simulink model "stewart_platform"  (R2019b)
settings: configuration reference "conf_simscape" (kept outside this file)
undefined symbols (not defined in the file): stewart, X, Y, Z
libraries: sm_lib x20, nesl_utility x1
settings Model: Creator=thomas  LastModifiedBy=thomas
settings ConfigSetRef: SourceName=conf_simscape  SourceLocation=Base Workspace

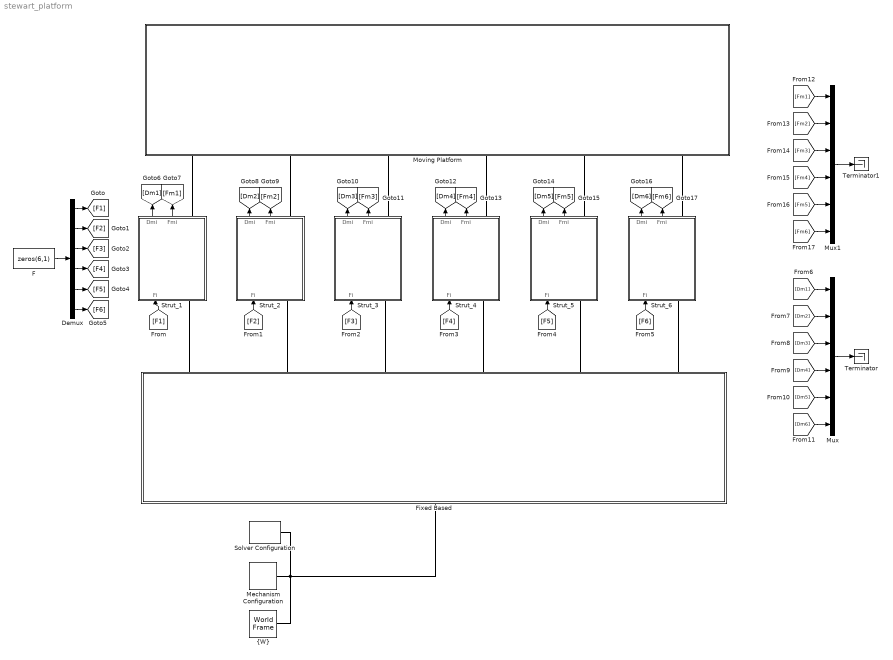
== system stewart_platform ==
  Demux : Demux  Outputs=6
  F : Constant  Value=zeros(6,1)
  Fixed Based : Subsystem
  Mechanism Configuration : sm_lib/Utilities/Mechanism Configuration  UniformGravity=Constant  GravityVector=[0 0 0]  GravityUnits=m/s^2  LinearizationDelta=0.001
  Moving Platform : Subsystem
  Mux : Mux  Inputs=6
  Mux1 : Mux  Inputs=6
  Solver Configuration : nesl_utility/Solver Configuration  PhysicalDomain=network_engine_domain  SubClassName=solver  LeftPortType=input  RightPortType=generic  Tones=[]  Harmonics=[]  SimulateNoise=off  Profile=off  UseLocalSampling=off  EnableSwitchedLinearOptims=on  FrequencyDomain=off  UseCCode=off  RelTol=0.001  AbsTol=1e-06  MinStep=1e-09  ToWorkspace=off  RevertToSquareIcSolve=off  NumHomotopyIterations=100  PhasorMode=off  PhasorModeNumHarmonics=1  DoDC=off  ResidualTolerance=1e-09  UseLocalSolver=off  LocalSolverChoice=NE_BACKWARD_EULER_ADVANCER  LocalSolverSampleTime=0.001  DoFixedCost=off  MaxNonlinIter=3  MaxModeIter=2  LinearAlgebra=auto  EquationFormulation=NE_TIME_EF  DelaysMemoryBudget=1024  AutomaticFiltering=on  FilteringTimeConstant=0.001  PartitionStorageMethod=AS_NEEDED  PartitionMemoryBudget=1024  PartitionMethod=ROBUST
  Strut_1 : Subsystem
      mask init:
      | i=1;
  Strut_2 : Subsystem
      mask init:
      | i=2;
  Strut_3 : Subsystem
      mask init:
      | i=3;
  Strut_4 : Subsystem
      mask init:
      | i=4;
  Strut_5 : Subsystem
      mask init:
      | i=5;
  Strut_6 : Subsystem
      mask init:
      | i=6;
  Terminator : Terminator
  Terminator1 : Terminator
  "{W}" : sm_lib/Frames and Transforms/World Frame
  wires:
  F/1 -> Demux/1
  Demux/1 -> [F1]
  Demux/2 -> [F2]
  [F1] -> Strut_1/1(Fi)
  Demux/3 -> [F3]
  Demux/4 -> [F4]
  Demux/5 -> [F5]
  Demux/6 -> [F6]
  [F2] -> Strut_2/1(Fi)
  [F4] -> Strut_4/1(Fi)
  [F5] -> Strut_5/1(Fi)
  [F6] -> Strut_6/1(Fi)
  Strut_1/1(Dmi) -> [Dm1]
  Strut_1/2(Fmi) -> [Fm1]
  Strut_2/2(Fmi) -> [Fm2]
  [F3] -> Strut_3/1(Fi)
  Strut_2/1(Dmi) -> [Dm2]
  Strut_3/1(Dmi) -> [Dm3]
  Strut_3/2(Fmi) -> [Fm3]
  Strut_4/1(Dmi) -> [Dm4]
  Strut_4/2(Fmi) -> [Fm4]
  Strut_5/1(Dmi) -> [Dm5]
  Strut_5/2(Fmi) -> [Fm5]
  Strut_6/1(Dmi) -> [Dm6]
  Strut_6/2(Fmi) -> [Fm6]
  [Dm2] -> Mux/2
  [Dm1] -> Mux/1
  [Dm3] -> Mux/3
  [Dm4] -> Mux/4
  [Dm5] -> Mux/5
  [Dm6] -> Mux/6
  Mux/1 -> Terminator/1
  [Fm6] -> Mux1/6
  [Fm5] -> Mux1/5
  [Fm1] -> Mux1/1
  [Fm2] -> Mux1/2
  [Fm3] -> Mux1/3
  [Fm4] -> Mux1/4
  Mux1/1 -> Terminator1/1
  connections:
  "{W}"/RConn1 -- Fixed Based/LConn1 -- Solver Configuration/RConn1 -- Mechanism Configuration/RConn1
  Fixed Based/RConn2 -- Strut_2/LConn1
  Fixed Based/RConn3 -- Strut_3/LConn1
  Fixed Based/RConn4 -- Strut_4/LConn1
  Fixed Based/RConn5 -- Strut_5/LConn1
  Fixed Based/RConn6 -- Strut_6/LConn1
  Strut_2/RConn1 -- Moving Platform/LConn2
  Strut_3/RConn1 -- Moving Platform/LConn3
  Strut_4/RConn1 -- Moving Platform/LConn4
  Strut_5/RConn1 -- Moving Platform/LConn5
  Strut_6/RConn1 -- Moving Platform/LConn6
  Strut_1/LConn1 -- Fixed Based/RConn1
  Strut_1/RConn1 -- Moving Platform/LConn1

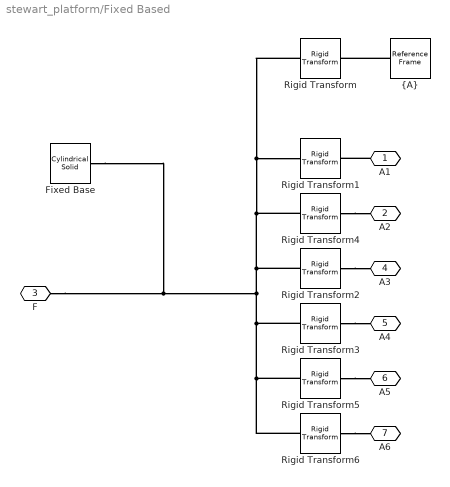
== system stewart_platform/Fixed Based ==
  Fixed Base : sm_lib/Body Elements/Cylindrical Solid  GraphicAmbientColor=[0.15 0.15 0.15 1.0]  BasedOnType=Density  CenterOfMass=[0 0 0]  CenterOfMassUnits=m  GraphicDiffuseColor=[0.5 0.5 0.5]  CylinderLength=10e-3  CylinderLengthUnits=m  CylinderRadius=100e-3  CylinderRadiusUnits=m  Density=1000  DensityUnits=kg/m^3  DoExposeReferenceFrame=off  GraphicEmissiveColor=[0.0 0.0 0.0 1.0]  ExportEntireGeometry=off  SerializedFrames=<Frames><Frame><Id>Frame1</Id><Value><Name>{F}</Name><Origin><Source>GeometricFeature</Source><FeatureName>bottom surface</FeatureName></Origin><PrimaryAxis><DefinedDirection>+Z</DefinedDirection><Source>ReferenceFrame</Source><SourceDirection>+Z</SourceDirection><FeatureName></FeatureName></PrimaryAxis><SecondaryAxis><DefinedDirection>+X</DefinedDirection><Source>ReferenceFrame</Source><SourceDirection>+X</SourceDirection><FeatureName></FeatureName></SecondaryAxis></Value></Frame></Frames>  MarkerShape=Sphere  MarkerSize=10  GraphicType=FromGeometry  InertiaType=CalculateFromGeometry  Mass=1  MassUnits=kg  MomentsOfInertia=[1 1 1]  MomentsOfInertiaUnits=kg*m^2  GraphicOpacity=1.0  ProductsOfInertia=[0 0 0]  ProductsOfInertiaUnits=kg*m^2  GraphicShininess=75  GraphicSpecularColor=[0.5 0.5 0.5 1.0]  GraphicVisPropType=SimpleVisualProperties
  Rigid Transform : sm_lib/Frames and Transforms/Rigid Transform  TranslationMethod=Cartesian  TranslationStandardOffset=0  TranslationLengthUnit=m  TranslationStandardAxis=+Z  TranslationCartesianOffset=stewart.FO_A  TranslationROffset=0  TranslationROffsetUnits=m  TranslationZOffset=0  TranslationZOffsetUnits=m  TranslationThetaOffset=0  TranslationThetaOffsetUnits=deg  RotationMethod=None  RotationAngleUnits=deg  RotationStandardAxis=+Z  RotationAngle=0.0  RotationArbitraryAxis=[0 0 1]  FollAlignAxisA=+X  BaseAlignAxisA=+Y  FollAlignAxisB=+Y  BaseAlignAxisB=+Z  RotationSequenceAxes=FollowerAxes  RotationSequence=XYX  RotationSequenceAngles=[0 0 0]  RotationSequenceAnglesUnits=deg  RotationMatrix=[1 0 0; 0 1 0; 0 0 1]
  Rigid Transform1 : sm_lib/Frames and Transforms/Rigid Transform  TranslationMethod=Cartesian  TranslationStandardOffset=0  TranslationLengthUnit=m  TranslationStandardAxis=+Z  TranslationCartesianOffset=stewart.Fa(:, 1)  TranslationROffset=0  TranslationROffsetUnits=m  TranslationZOffset=0  TranslationZOffsetUnits=m  TranslationThetaOffset=0  TranslationThetaOffsetUnits=deg  RotationMethod=RotationMatrix  RotationAngleUnits=deg  RotationStandardAxis=+Z  RotationAngle=0.0  RotationArbitraryAxis=[0 0 1]  FollAlignAxisA=+X  BaseAlignAxisA=+Y  FollAlignAxisB=+Y  BaseAlignAxisB=+Z  RotationSequenceAxes=FollowerAxes  RotationSequence=XYX  RotationSequenceAngles=[0 0 0]  RotationSequenceAnglesUnits=deg  RotationMatrix=stewart.FRa(:, :, 1)
  Rigid Transform2 : sm_lib/Frames and Transforms/Rigid Transform  TranslationMethod=Cartesian  TranslationStandardOffset=0  TranslationLengthUnit=m  TranslationStandardAxis=+Z  TranslationCartesianOffset=stewart.Fa(:, 3)  TranslationROffset=0  TranslationROffsetUnits=m  TranslationZOffset=0  TranslationZOffsetUnits=m  TranslationThetaOffset=0  TranslationThetaOffsetUnits=deg  RotationMethod=RotationMatrix  RotationAngleUnits=deg  RotationStandardAxis=+Z  RotationAngle=0.0  RotationArbitraryAxis=[0 0 1]  FollAlignAxisA=+X  BaseAlignAxisA=+Y  FollAlignAxisB=+Y  BaseAlignAxisB=+Z  RotationSequenceAxes=FollowerAxes  RotationSequence=XYX  RotationSequenceAngles=[0 0 0]  RotationSequenceAnglesUnits=deg  RotationMatrix=stewart.FRa(:, :, 3)
  Rigid Transform3 : sm_lib/Frames and Transforms/Rigid Transform  TranslationMethod=Cartesian  TranslationStandardOffset=0  TranslationLengthUnit=m  TranslationStandardAxis=+Z  TranslationCartesianOffset=stewart.Fa(:, 4)  TranslationROffset=0  TranslationROffsetUnits=m  TranslationZOffset=0  TranslationZOffsetUnits=m  TranslationThetaOffset=0  TranslationThetaOffsetUnits=deg  RotationMethod=RotationMatrix  RotationAngleUnits=deg  RotationStandardAxis=+Z  RotationAngle=0.0  RotationArbitraryAxis=[0 0 1]  FollAlignAxisA=+X  BaseAlignAxisA=+Y  FollAlignAxisB=+Y  BaseAlignAxisB=+Z  RotationSequenceAxes=FollowerAxes  RotationSequence=XYX  RotationSequenceAngles=[0 0 0]  RotationSequenceAnglesUnits=deg  RotationMatrix=stewart.FRa(:, :, 4)
  Rigid Transform4 : sm_lib/Frames and Transforms/Rigid Transform  TranslationMethod=Cartesian  TranslationStandardOffset=0  TranslationLengthUnit=m  TranslationStandardAxis=+Z  TranslationCartesianOffset=stewart.Fa(:, 2)  TranslationROffset=0  TranslationROffsetUnits=m  TranslationZOffset=0  TranslationZOffsetUnits=m  TranslationThetaOffset=0  TranslationThetaOffsetUnits=deg  RotationMethod=RotationMatrix  RotationAngleUnits=deg  RotationStandardAxis=+Z  RotationAngle=0.0  RotationArbitraryAxis=[0 0 1]  FollAlignAxisA=+X  BaseAlignAxisA=+Y  FollAlignAxisB=+Y  BaseAlignAxisB=+Z  RotationSequenceAxes=FollowerAxes  RotationSequence=XYX  RotationSequenceAngles=[0 0 0]  RotationSequenceAnglesUnits=deg  RotationMatrix=stewart.FRa(:, :, 2)
  Rigid Transform5 : sm_lib/Frames and Transforms/Rigid Transform  TranslationMethod=Cartesian  TranslationStandardOffset=0  TranslationLengthUnit=m  TranslationStandardAxis=+Z  TranslationCartesianOffset=stewart.Fa(:, 5)  TranslationROffset=0  TranslationROffsetUnits=m  TranslationZOffset=0  TranslationZOffsetUnits=m  TranslationThetaOffset=0  TranslationThetaOffsetUnits=deg  RotationMethod=RotationMatrix  RotationAngleUnits=deg  RotationStandardAxis=+Z  RotationAngle=0.0  RotationArbitraryAxis=[0 0 1]  FollAlignAxisA=+X  BaseAlignAxisA=+Y  FollAlignAxisB=+Y  BaseAlignAxisB=+Z  RotationSequenceAxes=FollowerAxes  RotationSequence=XYX  RotationSequenceAngles=[0 0 0]  RotationSequenceAnglesUnits=deg  RotationMatrix=stewart.FRa(:, :, 5)
  Rigid Transform6 : sm_lib/Frames and Transforms/Rigid Transform  TranslationMethod=Cartesian  TranslationStandardOffset=0  TranslationLengthUnit=m  TranslationStandardAxis=+Z  TranslationCartesianOffset=stewart.Fa(:, 6)  TranslationROffset=0  TranslationROffsetUnits=m  TranslationZOffset=0  TranslationZOffsetUnits=m  TranslationThetaOffset=0  TranslationThetaOffsetUnits=deg  RotationMethod=RotationMatrix  RotationAngleUnits=deg  RotationStandardAxis=+Z  RotationAngle=0.0  RotationArbitraryAxis=[0 0 1]  FollAlignAxisA=+X  BaseAlignAxisA=+Y  FollAlignAxisB=+Y  BaseAlignAxisB=+Z  RotationSequenceAxes=FollowerAxes  RotationSequence=XYX  RotationSequenceAngles=[0 0 0]  RotationSequenceAnglesUnits=deg  RotationMatrix=stewart.FRa(:, :, 6)
  "{A}" : sm_lib/Frames and Transforms/Reference Frame
  A1 : PMIOPort  Side=Right
  A2 : PMIOPort  Port=2  Side=Right
  F : PMIOPort  Port=3  Side=Left
  A3 : PMIOPort  Port=4  Side=Right
  A4 : PMIOPort  Port=5  Side=Right
  A5 : PMIOPort  Port=6  Side=Right
  A6 : PMIOPort  Port=7  Side=Right
  connections:
  Rigid Transform4/RConn1 -- A2/RConn1
  "{A}"/RConn1 -- Rigid Transform/RConn1
  A1/RConn1 -- Rigid Transform1/RConn1
  Rigid Transform/LConn1 -- Rigid Transform1/LConn1 -- Rigid Transform6/LConn1 -- Rigid Transform5/LConn1 -- Rigid Transform3/LConn1 -- F/RConn1 -- Fixed Base/LConn1 -- Rigid Transform2/LConn1 -- Rigid Transform4/LConn1
  Rigid Transform2/RConn1 -- A3/RConn1
  Rigid Transform3/RConn1 -- A4/RConn1
  Rigid Transform5/RConn1 -- A5/RConn1
  Rigid Transform6/RConn1 -- A6/RConn1

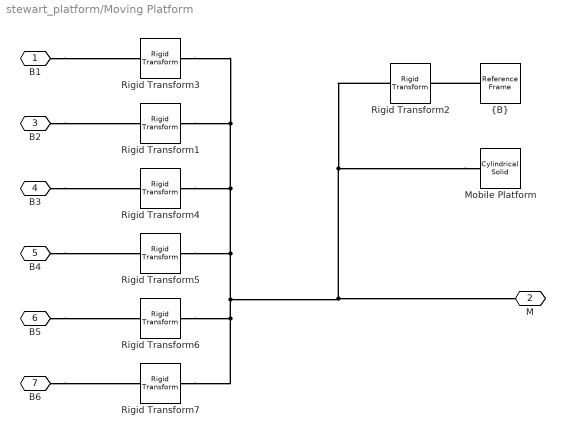
== system stewart_platform/Moving Platform ==
  Mobile Platform : sm_lib/Body Elements/Cylindrical Solid  GraphicAmbientColor=[0.15 0.15 0.15 1.0]  BasedOnType=Density  CenterOfMass=[0 0 0]  CenterOfMassUnits=m  GraphicDiffuseColor=[0.5 0.5 0.5]  CylinderLength=10e-3  CylinderLengthUnits=m  CylinderRadius=100e-3  CylinderRadiusUnits=m  Density=1000  DensityUnits=kg/m^3  DoExposeReferenceFrame=off  GraphicEmissiveColor=[0.0 0.0 0.0 1.0]  ExportEntireGeometry=off  SerializedFrames=<Frames><Frame><Id>Frame1</Id><Value><Name>{M}</Name><Origin><Source>GeometricFeature</Source><FeatureName>top surface</FeatureName></Origin><PrimaryAxis><DefinedDirection>+Z</DefinedDirection><Source>ReferenceFrame</Source><SourceDirection>+Z</SourceDirection><FeatureName></FeatureName></PrimaryAxis><SecondaryAxis><DefinedDirection>+X</DefinedDirection><Source>ReferenceFrame</Source><SourceDirection>+X</SourceDirection><FeatureName></FeatureName></SecondaryAxis></Value></Frame></Frames>  MarkerShape=Sphere  MarkerSize=10  GraphicType=FromGeometry  InertiaType=CalculateFromGeometry  Mass=1  MassUnits=kg  MomentsOfInertia=[1 1 1]  MomentsOfInertiaUnits=kg*m^2  GraphicOpacity=1.0  ProductsOfInertia=[0 0 0]  ProductsOfInertiaUnits=kg*m^2  GraphicShininess=75  GraphicSpecularColor=[0.5 0.5 0.5 1.0]  GraphicVisPropType=SimpleVisualProperties
  Rigid Transform1 : sm_lib/Frames and Transforms/Rigid Transform  TranslationMethod=Cartesian  TranslationStandardOffset=0  TranslationLengthUnit=m  TranslationStandardAxis=+Z  TranslationCartesianOffset=stewart.Mb(:, 2)  TranslationROffset=0  TranslationROffsetUnits=m  TranslationZOffset=0  TranslationZOffsetUnits=m  TranslationThetaOffset=0  TranslationThetaOffsetUnits=deg  RotationMethod=RotationMatrix  RotationAngleUnits=deg  RotationStandardAxis=+Z  RotationAngle=0.0  RotationArbitraryAxis=[0 0 1]  FollAlignAxisA=+X  BaseAlignAxisA=+Y  FollAlignAxisB=+Y  BaseAlignAxisB=+Z  RotationSequenceAxes=FollowerAxes  RotationSequence=XYX  RotationSequenceAngles=[0 0 0]  RotationSequenceAnglesUnits=deg  RotationMatrix=stewart.MRb(:, :, 2)
  Rigid Transform2 : sm_lib/Frames and Transforms/Rigid Transform  TranslationMethod=Cartesian  TranslationStandardOffset=0  TranslationLengthUnit=m  TranslationStandardAxis=+Z  TranslationCartesianOffset=stewart.MO_B  TranslationROffset=0  TranslationROffsetUnits=m  TranslationZOffset=0  TranslationZOffsetUnits=m  TranslationThetaOffset=0  TranslationThetaOffsetUnits=deg  RotationMethod=None  RotationAngleUnits=deg  RotationStandardAxis=+Z  RotationAngle=0.0  RotationArbitraryAxis=[0 0 1]  FollAlignAxisA=+X  BaseAlignAxisA=+Y  FollAlignAxisB=+Y  BaseAlignAxisB=+Z  RotationSequenceAxes=FollowerAxes  RotationSequence=XYX  RotationSequenceAngles=[0 0 0]  RotationSequenceAnglesUnits=deg  RotationMatrix=[1 0 0; 0 1 0; 0 0 1]
  Rigid Transform3 : sm_lib/Frames and Transforms/Rigid Transform  TranslationMethod=Cartesian  TranslationStandardOffset=0  TranslationLengthUnit=m  TranslationStandardAxis=+Z  TranslationCartesianOffset=stewart.Mb(:, 1)  TranslationROffset=0  TranslationROffsetUnits=m  TranslationZOffset=0  TranslationZOffsetUnits=m  TranslationThetaOffset=0  TranslationThetaOffsetUnits=deg  RotationMethod=RotationMatrix  RotationAngleUnits=deg  RotationStandardAxis=+Z  RotationAngle=0.0  RotationArbitraryAxis=[0 0 1]  FollAlignAxisA=+X  BaseAlignAxisA=+Y  FollAlignAxisB=+Y  BaseAlignAxisB=+Z  RotationSequenceAxes=FollowerAxes  RotationSequence=XYX  RotationSequenceAngles=[0 0 0]  RotationSequenceAnglesUnits=deg  RotationMatrix=stewart.MRb(:, :, 1)
  Rigid Transform4 : sm_lib/Frames and Transforms/Rigid Transform  TranslationMethod=Cartesian  TranslationStandardOffset=0  TranslationLengthUnit=m  TranslationStandardAxis=+Z  TranslationCartesianOffset=stewart.Mb(:, 3)  TranslationROffset=0  TranslationROffsetUnits=m  TranslationZOffset=0  TranslationZOffsetUnits=m  TranslationThetaOffset=0  TranslationThetaOffsetUnits=deg  RotationMethod=RotationMatrix  RotationAngleUnits=deg  RotationStandardAxis=+Z  RotationAngle=0.0  RotationArbitraryAxis=[0 0 1]  FollAlignAxisA=+X  BaseAlignAxisA=+Y  FollAlignAxisB=+Y  BaseAlignAxisB=+Z  RotationSequenceAxes=FollowerAxes  RotationSequence=XYX  RotationSequenceAngles=[0 0 0]  RotationSequenceAnglesUnits=deg  RotationMatrix=stewart.MRb(:, :, 3)
  Rigid Transform5 : sm_lib/Frames and Transforms/Rigid Transform  TranslationMethod=Cartesian  TranslationStandardOffset=0  TranslationLengthUnit=m  TranslationStandardAxis=+Z  TranslationCartesianOffset=stewart.Mb(:, 4)  TranslationROffset=0  TranslationROffsetUnits=m  TranslationZOffset=0  TranslationZOffsetUnits=m  TranslationThetaOffset=0  TranslationThetaOffsetUnits=deg  RotationMethod=RotationMatrix  RotationAngleUnits=deg  RotationStandardAxis=+Z  RotationAngle=0.0  RotationArbitraryAxis=[0 0 1]  FollAlignAxisA=+X  BaseAlignAxisA=+Y  FollAlignAxisB=+Y  BaseAlignAxisB=+Z  RotationSequenceAxes=FollowerAxes  RotationSequence=XYX  RotationSequenceAngles=[0 0 0]  RotationSequenceAnglesUnits=deg  RotationMatrix=stewart.MRb(:, :, 4)
  Rigid Transform6 : sm_lib/Frames and Transforms/Rigid Transform  TranslationMethod=Cartesian  TranslationStandardOffset=0  TranslationLengthUnit=m  TranslationStandardAxis=+Z  TranslationCartesianOffset=stewart.Mb(:, 5)  TranslationROffset=0  TranslationROffsetUnits=m  TranslationZOffset=0  TranslationZOffsetUnits=m  TranslationThetaOffset=0  TranslationThetaOffsetUnits=deg  RotationMethod=RotationMatrix  RotationAngleUnits=deg  RotationStandardAxis=+Z  RotationAngle=0.0  RotationArbitraryAxis=[0 0 1]  FollAlignAxisA=+X  BaseAlignAxisA=+Y  FollAlignAxisB=+Y  BaseAlignAxisB=+Z  RotationSequenceAxes=FollowerAxes  RotationSequence=XYX  RotationSequenceAngles=[0 0 0]  RotationSequenceAnglesUnits=deg  RotationMatrix=stewart.MRb(:, :, 5)
  Rigid Transform7 : sm_lib/Frames and Transforms/Rigid Transform  TranslationMethod=Cartesian  TranslationStandardOffset=0  TranslationLengthUnit=m  TranslationStandardAxis=+Z  TranslationCartesianOffset=stewart.Mb(:, 6)  TranslationROffset=0  TranslationROffsetUnits=m  TranslationZOffset=0  TranslationZOffsetUnits=m  TranslationThetaOffset=0  TranslationThetaOffsetUnits=deg  RotationMethod=RotationMatrix  RotationAngleUnits=deg  RotationStandardAxis=+Z  RotationAngle=0.0  RotationArbitraryAxis=[0 0 1]  FollAlignAxisA=+X  BaseAlignAxisA=+Y  FollAlignAxisB=+Y  BaseAlignAxisB=+Z  RotationSequenceAxes=FollowerAxes  RotationSequence=XYX  RotationSequenceAngles=[0 0 0]  RotationSequenceAnglesUnits=deg  RotationMatrix=stewart.MRb(:, :, 6)
  "{B}" : sm_lib/Frames and Transforms/Reference Frame
  B1 : PMIOPort  Side=Left
  M : PMIOPort  Port=2  Side=Right
  B2 : PMIOPort  Port=3  Side=Left
  B3 : PMIOPort  Port=4  Side=Left
  B4 : PMIOPort  Port=5  Side=Left
  B5 : PMIOPort  Port=6  Side=Left
  B6 : PMIOPort  Port=7  Side=Left
  connections:
  Mobile Platform/LConn1 -- Rigid Transform5/LConn1 -- Rigid Transform4/LConn1 -- Rigid Transform1/LConn1 -- Rigid Transform3/LConn1 -- Rigid Transform6/LConn1 -- Rigid Transform7/LConn1 -- M/RConn1 -- Rigid Transform2/LConn1
  B1/RConn1 -- Rigid Transform3/RConn1
  "{B}"/RConn1 -- Rigid Transform2/RConn1
  B2/RConn1 -- Rigid Transform1/RConn1
  B3/RConn1 -- Rigid Transform4/RConn1
  B4/RConn1 -- Rigid Transform5/RConn1
  B5/RConn1 -- Rigid Transform6/RConn1
  B6/RConn1 -- Rigid Transform7/RConn1

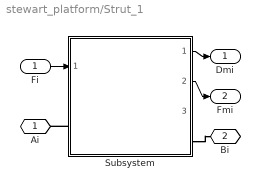
== system stewart_platform/Strut_1 ==
  Fi : Inport
  Subsystem : Subsystem  VariantControl=with_sensors  ReferencedSubsystem=stewart_strut
  Ai : PMIOPort  Side=Left
  Bi : PMIOPort  Port=2  Side=Right
  Dmi : Outport
  Fmi : Outport  Port=2
  wires:
  Subsystem/1 -> Dmi/1
  Subsystem/2 -> Fmi/1
  Fi/1 -> Subsystem/1
  connections:
  Subsystem/LConn1 -- Ai/RConn1
  Subsystem/RConn1 -- Bi/RConn1

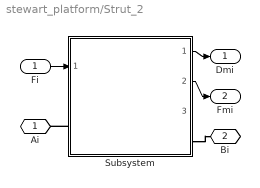
== system stewart_platform/Strut_2 ==
  Fi : Inport
  Subsystem : Subsystem  VariantControl=with_sensors  ReferencedSubsystem=stewart_strut
  Ai : PMIOPort  Side=Left
  Bi : PMIOPort  Port=2  Side=Right
  Dmi : Outport
  Fmi : Outport  Port=2
  wires:
  Fi/1 -> Subsystem/1
  Subsystem/2 -> Fmi/1
  Subsystem/1 -> Dmi/1
  connections:
  Subsystem/RConn1 -- Bi/RConn1
  Subsystem/LConn1 -- Ai/RConn1

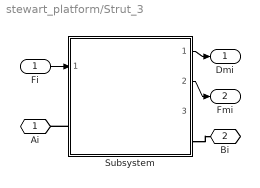
== system stewart_platform/Strut_3 ==
  Fi : Inport
  Subsystem : Subsystem  VariantControl=with_sensors  ReferencedSubsystem=stewart_strut
  Ai : PMIOPort  Side=Left
  Bi : PMIOPort  Port=2  Side=Right
  Dmi : Outport
  Fmi : Outport  Port=2
  wires:
  Subsystem/1 -> Dmi/1
  Subsystem/2 -> Fmi/1
  Fi/1 -> Subsystem/1
  connections:
  Subsystem/LConn1 -- Ai/RConn1
  Subsystem/RConn1 -- Bi/RConn1

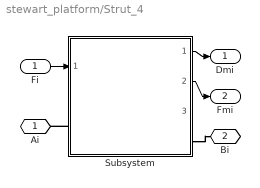
== system stewart_platform/Strut_4 ==
  Fi : Inport
  Subsystem : Subsystem  VariantControl=with_sensors  ReferencedSubsystem=stewart_strut
  Ai : PMIOPort  Side=Left
  Bi : PMIOPort  Port=2  Side=Right
  Dmi : Outport
  Fmi : Outport  Port=2
  wires:
  Fi/1 -> Subsystem/1
  Subsystem/2 -> Fmi/1
  Subsystem/1 -> Dmi/1
  connections:
  Subsystem/RConn1 -- Bi/RConn1
  Subsystem/LConn1 -- Ai/RConn1

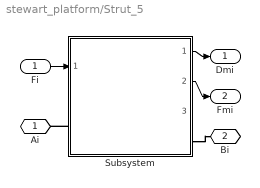
== system stewart_platform/Strut_5 ==
  Fi : Inport
  Subsystem : Subsystem  VariantControl=with_sensors  ReferencedSubsystem=stewart_strut
  Ai : PMIOPort  Side=Left
  Bi : PMIOPort  Port=2  Side=Right
  Dmi : Outport
  Fmi : Outport  Port=2
  wires:
  Subsystem/1 -> Dmi/1
  Subsystem/2 -> Fmi/1
  Fi/1 -> Subsystem/1
  connections:
  Subsystem/LConn1 -- Ai/RConn1
  Subsystem/RConn1 -- Bi/RConn1

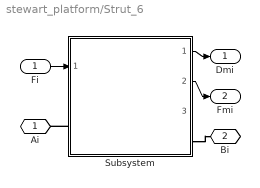
== system stewart_platform/Strut_6 ==
  Fi : Inport
  Subsystem : Subsystem  VariantControl=with_sensors  ReferencedSubsystem=stewart_strut
  Ai : PMIOPort  Side=Left
  Bi : PMIOPort  Port=2  Side=Right
  Dmi : Outport
  Fmi : Outport  Port=2
  wires:
  Fi/1 -> Subsystem/1
  Subsystem/2 -> Fmi/1
  Subsystem/1 -> Dmi/1
  connections:
  Subsystem/RConn1 -- Bi/RConn1
  Subsystem/LConn1 -- Ai/RConn1
